simulink model "HeadwayNonLinearFede"  (R2020a)
settings: Solver=VariableStepAuto  StartTime=0.0  StopTime=60  RelTol=1e-3
values from neighbouring files (symbols this model uses):
  K = lqr(A,B,Q,R)    [HeadwayFede.m]
  xe = [iq1_ref; id1_ref; iq2_ref; id2_ref; v_ref]    [HeadwayFede.m]
settings Model: Creator=Federico  LastModifiedBy=Federico

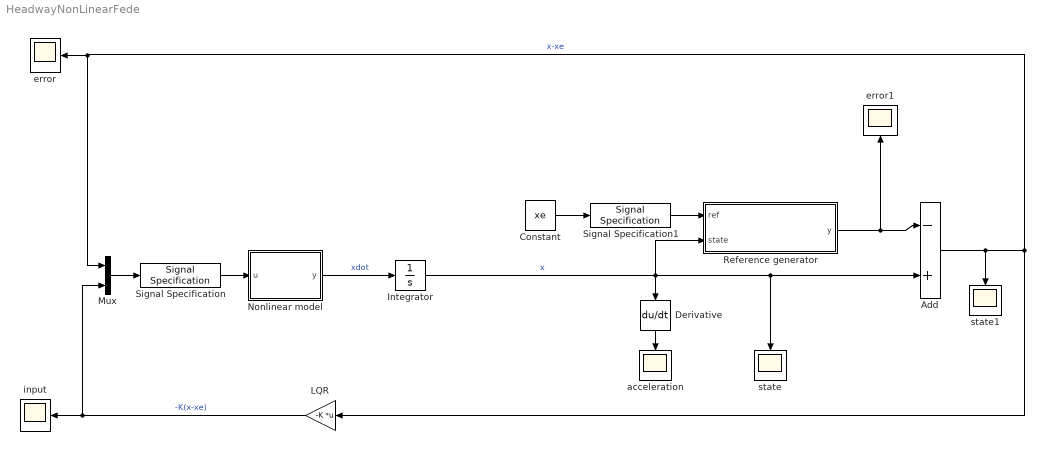
== system HeadwayNonLinearFede ==
  Add : Sum  Inputs=-+
  Constant : Constant  Value=xe
  Derivative : Derivative
  Integrator : Integrator  InitialCondition=[0;0;0;0;0]
  LQR : Gain  Gain=-K  Multiplication=Matrix(K*u)
  Mux : Mux  Inputs=2
  Nonlinear model : MATLAB Function  TreatAsAtomicUnit=on
  Reference generator : MATLAB Function  TreatAsAtomicUnit=on
  Signal Specification : SignalSpecification  Dimensions=9
  Signal Specification1 : SignalSpecification  Dimensions=5
  acceleration : Scope
  error : Scope
  error1 : Scope
  input : Scope
  state : Scope
  state1 : Scope
  wires:
  Integrator/1 -> Reference generator/2(state), Add/2, state/1, Derivative/1  "x"
  Mux/1 -> Signal Specification/1
  Add/1 -> state1/1, Mux/1, error/1, LQR/1  "x-xe"
  LQR/1 -> Mux/2, input/1  "-K(x-xe)"
  Signal Specification/1 -> Nonlinear model/1(u)
  Derivative/1 -> acceleration/1
  Nonlinear model/1(y) -> Integrator/1  "xdot"
  Reference generator/1(y) -> error1/1, Add/1
  Signal Specification1/1 -> Reference generator/1(ref)
  Constant/1 -> Signal Specification1/1

== matlab function HeadwayNonLinearFede/Reference generator ==
  data: y output; ref input; state input
function y = fcn(ref, state)

y = zeros(5,1);

%current references
y(1) = ref(1);
y(2) = ref(2);
y(3) = ref(3);
y(4) = ref(4);

y(5) = state(5);


v_ref = ref(5); % velocity v_reference
tollerance = 0.1; %needed to obtain a good final beaviour
accFactor = 0.1; %with this you can change the slope of the velocity and so the acceleration

%Speed ramp profile
if y(5) < v_ref - tollerance
    y(5)=(y(5)+accFactor);
elseif y(5) > v_ref + tollerance
    y(5)=(y(5)-accFactor);
else
    y(5)=v_ref;
end

== matlab function HeadwayNonLinearFede/Nonlinear model ==
  data: u input; y output
function y = fcn(u)
% u has 9 elements: the first five are the states and the last five the
% inputs

z=1; % nominal z
i_e=1; % nominal current which provide nominal z
R=1;
Ld=1;
Lq=1;
M=1;%mutual inductance stator rotor
tau=1;
p=3;% poli !
m=1;% mass 
rho=1;
S=1;
Cd=1;


iq1 = u(1);
id1 = u(2);
iq2 = u(3);
id2 = u(4);
v   = u(5);
Vq1 = u(6);
Vd1 = u(7);
Vq2 = u(8);
Vd2 = u(9);

iq1_dot = -(R/Lq)*iq1 - (Ld/Lq)*((M/Ld)*i_e + id1)*v*pi/tau + Vq1/Lq ;
iq2_dot = -(R/Lq)*iq2 - (Ld/Lq)*((M/Ld)*i_e + id2)*v*pi/tau + Vq2/Lq ;

id1_dot = -(R/Ld)*id1 + (Lq/Ld)*(iq1)*v*pi/tau + Vd1/Ld ;
id2_dot = -(R/Ld)*id2 + (Lq/Ld)*(iq2)*v*pi/tau + Vd2/Ld ;

Fx1 = (3/2)*(pi/tau)*(Ld*((M/Ld)*i_e) + (Ld-Lq)*id1)*iq1;
Fx2 = (3/2)*(pi/tau)*(Ld*((M/Ld)*i_e) + (Ld-Lq)*id2)*iq2;

v_dot = (1/m)*(p*Fx1 + p*Fx2 -(rho*S*Cd/2)*v^2);

y = [iq1_dot; id1_dot; iq2_dot; id2_dot; v_dot];
